simulink model "pidusingopamp"  (R2015a)
settings: Solver=ode15s  StartTime=0.0  StopTime=0.005  MaxStep=0.00002  RelTol=1e-3
libraries: fl_lib x10, nesl_utility x3
Description:
  | Differentiator
  | 
  | This model shows a differentiator, such as might be used as part
  | of a PID controller. It also illustrates how numerical simulation issues
  | can arise in some idealized circuits. The model runs with the
  | capacitor series parasitic resistance set to its default value of 1e-6
  | Ohms. Setting it to zero results in a warning and a very slow
  | simulation. See the User's Guide for further information.
  | 
  | 
  | Copyright 2008-2015 The MathWorks, Inc.
settings Model: ExtModeAutoUpdateStatusClock=off  Creator=MathWorks  LastModifiedBy=91703
settings DataIOCC: SignalLoggingSaveFormat=ModelDataLogs
settings OptimizationCC: ExpressionDepthLimit=2147483647  InitFltsAndDblsToZero=on
settings DebuggingCC: SaveWithParameterizedLinksMsg=none  UnderspecifiedInitializationDetection=Classic  MergeDetectMultiDrivingBlocksExec=none  SignalResolutionControl=TryResolveAllWithWarning  SolverPrmCheckMsg=warning  FcnCallInpInsideContextMsg=UseLocalSettings  StateNameClashWarn=warning
settings GRTTargetCC: TargetFcnLib=ansi_tfl_tmw.mat  CombineOutputUpdateFcns=off  GRTInterface=on

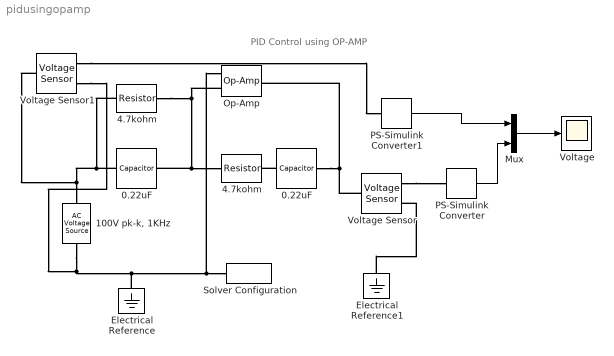
== system pidusingopamp ==
  note: PID Control using OP-AMP
  0.22uF : fl_lib/Electrical/Electrical Elements/Capacitor  c=0.22 uF  r=1e-6 Ohm  g=0 1/Ohm  i_specify=off  i_priority=High  i=0 A  v_specify=off  v_priority=High  v=0 V  vc_specify=on  vc_priority=High  vc=0 V
  "0.22uF " : fl_lib/Electrical/Electrical Elements/Capacitor  c=0.22 uF  r=1e-6 Ohm  g=0 1/Ohm  i_specify=off  i_priority=High  i=0 A  v_specify=off  v_priority=High  v=0 V  vc_specify=on  vc_priority=High  vc=0 V
  "100V pk-k, 1KHz" : fl_lib/Electrical/Electrical Sources/AC Voltage Source  amp=50 V  shift=0 deg  frequency=1000 Hz  omega=0 rad/s
  4.7kohm : fl_lib/Electrical/Electrical Elements/Resistor  R=4700 Ohm  i_specify=off  i_priority=High  i=0 A  v_specify=off  v_priority=High  v=0 V
  "4.7kohm " : fl_lib/Electrical/Electrical Elements/Resistor  R=4700 Ohm  i_specify=off  i_priority=High  i=0 A  v_specify=off  v_priority=High  v=0 V
  Electrical Reference : fl_lib/Electrical/Electrical Elements/Electrical Reference
  Electrical Reference1 : fl_lib/Electrical/Electrical Elements/Electrical Reference
  Mux : Mux  Inputs=2
  Op-Amp : fl_lib/Electrical/Electrical Elements/Op-Amp  outI_specify=off  outI_priority=High  outI=0 A
  PS-Simulink Converter : nesl_utility/PS-Simulink Converter  PhysicalDomain=network_engine_domain  SubClassName=ps_output  LeftPortType=input  RightPortType=output  PseudoPeriodic=off  Frequencies=[]  Unit=1  AffineConversion=off
  PS-Simulink Converter1 : nesl_utility/PS-Simulink Converter  PhysicalDomain=network_engine_domain  SubClassName=ps_output  LeftPortType=input  RightPortType=output  PseudoPeriodic=off  Frequencies=[]  Unit=1  AffineConversion=off
  Solver Configuration : nesl_utility/Solver Configuration  PhysicalDomain=network_engine_domain  SubClassName=solver  LeftPortType=input  RightPortType=generic  Accelerate=off  Tones=[]  Harmonics=[]  SimulateNoise=off  Profile=off  UseLocalSampling=off  EnableSwitchedLinearOptims=on  FrequencyDomain=off  UseCCode=off  RelTol=0.001  AbsTol=1e-06  MinStep=1e-09  ToWorkspace=off  RevertToSquareIcSolve=off  NumHomotopyIterations=100  DoDC=off  ResidualTolerance=1e-9  UseLocalSolver=off  LocalSolverChoice=NE_BACKWARD_EULER_ADVANCER  LocalSolverSampleTime=.001  DoFixedCost=off  MaxNonlinIter=3  MaxModeIter=2  LinearAlgebra=Sparse  DelaysMemoryBudget=1024  AutomaticFiltering=on  FilteringTimeConstant=0.001
  Voltage : Scope
      settings: YMin=-2  YMax=2  SaveName=ScopeData4
  Voltage Sensor : fl_lib/Electrical/Electrical Sensors/Voltage Sensor
  Voltage Sensor1 : fl_lib/Electrical/Electrical Sensors/Voltage Sensor
  wires:
  Mux/1 -> Voltage/1
  PS-Simulink Converter1/1 -> Mux/1
  PS-Simulink Converter/1 -> Mux/2
  connections:
  Voltage Sensor1/RConn2 -- "100V pk-k, 1KHz"/RConn1 -- Electrical Reference/LConn1 -- Op-Amp/LConn1 -- Solver Configuration/RConn1
  0.22uF/LConn1 -- "4.7kohm "/LConn1 -- Voltage Sensor1/LConn1 -- "100V pk-k, 1KHz"/LConn1
  0.22uF/RConn1 -- "4.7kohm "/RConn1 -- Op-Amp/LConn2 -- 4.7kohm/LConn1
  Voltage Sensor/LConn1 -- "0.22uF "/RConn1 -- Op-Amp/RConn1
  Electrical Reference1/LConn1 -- Voltage Sensor/RConn2
  Voltage Sensor/RConn1 -- PS-Simulink Converter/LConn1
  "0.22uF "/LConn1 -- 4.7kohm/RConn1
  Voltage Sensor1/RConn1 -- PS-Simulink Converter1/LConn1
